simulink model "aurea"  (R2021b)
settings: Solver=VariableStepAuto  StartTime=0.0  StopTime=1.0  RelTol=1e-3
settings Model: PauseTimes=1  Creator=tormena  LastModifiedBy=tormena

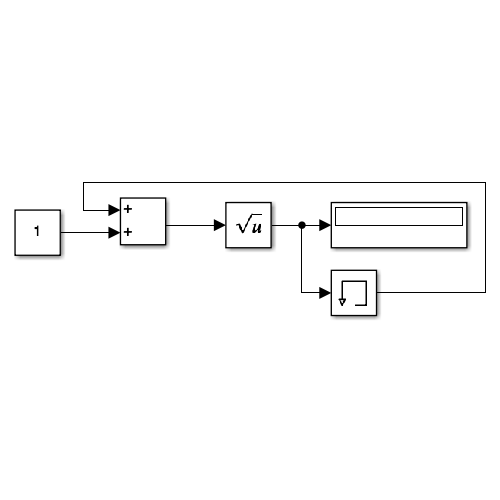
[thumbnail: Simulink's stored preview of the top-level diagram]
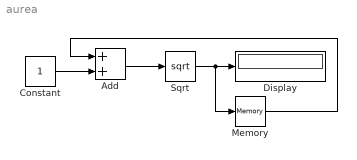
== system aurea ==
  Add : Sum
  Constant : Constant
  Display : Display
  Memory : Memory  InitialCondition=-1  InheritSampleTime=on
  Sqrt : Sqrt  SaturateOnIntegerOverflow=on
  wires:
  Sqrt/1 -> Memory/1, Display/1
  Memory/1 -> Add/1
  Constant/1 -> Add/2
  Add/1 -> Sqrt/1
